simulink model "TCP40_ON_OFF"  (Simulink 8.1)
settings: Solver=ode45  StartTime=0.0  StopTime=150  RelTol=1e-3
settings Model: Creator=cslui  LastModifiedBy=tohoanglinh
settings OptimizationCC: BlockReduction=off  BooleanDataType=off  ExpressionDepthLimit=128
settings DebuggingCC: SaveWithParameterizedLinksMsg=none  SignalResolutionControl=TryResolveAllWithWarning  SolverPrmCheckMsg=none  MultiTaskDSMMsg=warning  MultiTaskCondExecSysMsg=none  FcnCallInpInsideContextMsg=EnableAllAsError  StrictBusMsg=None
settings HardwareCC: TargetUnknown=on
settings RTWCC: IncludeERTFirstTime=on

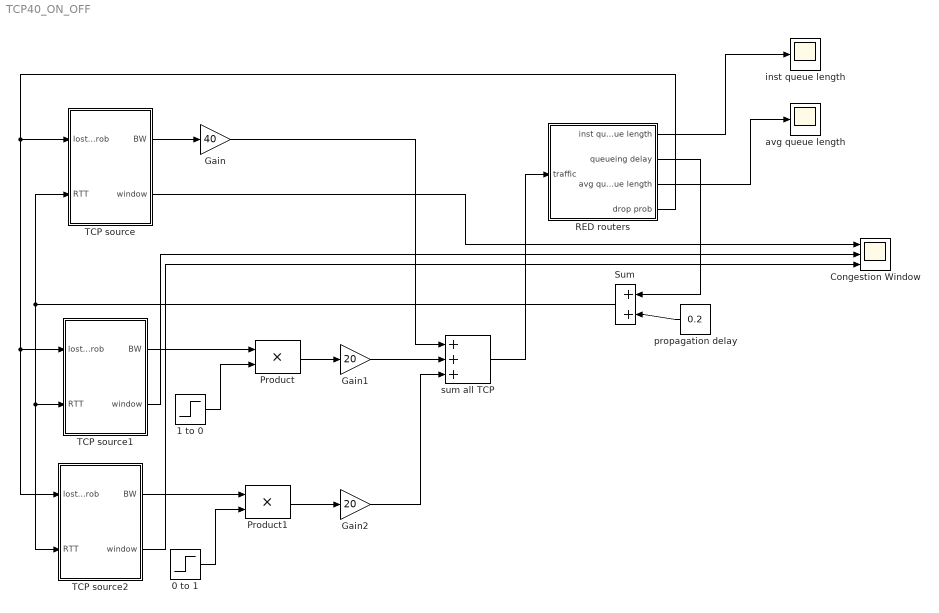
== system TCP40_ON_OFF ==
  0 to 1 : Step  Time=120  SampleTime=0
  1 to 0 : Step  Time=70  Before=1  After=0  SampleTime=0
  "Congestion Window " : Scope  NumInputPorts=3
      settings: YMin=0~-5~-5  YMax=30~5~5  SaveName=ScopeData2
  Gain : Gain  Gain=40  SaturateOnIntegerOverflow=on  OutDataTypeStr=Inherit: Same as input  ParamDataTypeStr=Inherit: Same as input
  Gain1 : Gain  Gain=20  SaturateOnIntegerOverflow=on  OutDataTypeStr=Inherit: Same as input  ParamDataTypeStr=Inherit: Same as input
  Gain2 : Gain  Gain=20  SaturateOnIntegerOverflow=on  OutDataTypeStr=Inherit: Same as input  ParamDataTypeStr=Inherit: Same as input
  Product : Product  SaturateOnIntegerOverflow=on  RndMeth=Zero  InputSameDT=on  OutDataTypeStr=Inherit: Same as first input
  Product1 : Product  SaturateOnIntegerOverflow=on  RndMeth=Zero  InputSameDT=on  OutDataTypeStr=Inherit: Same as first input
  RED routers : Subsystem  mask{C=1310}
      mask prompts: C "Router Capacity"
  Sum : Sum  Inputs=+|+  InputSameDT=on  OutDataTypeStr=Inherit: Same as first input
  TCP source : Subsystem
  TCP source1 : Subsystem
  TCP source2 : Subsystem
  avg queue length : Scope
      settings: YMin=0  YMax=800
  inst queue length : Scope
      settings: YMin=0  YMax=1000
  propagation delay : Constant  Value=0.2
  sum all TCP : Sum  Inputs=+|+|+  SaturateOnIntegerOverflow=on  InputSameDT=on  OutDataTypeStr=Inherit: Same as first input
  wires:
  TCP source/1(BW) -> Gain/1
  RED routers/2(queueing delay) -> Sum/1
  propagation delay/1 -> Sum/2
  Sum/1 -> TCP source/2(RTT), TCP source1/2(RTT), TCP source2/2(RTT)
  RED routers/4(drop prob) -> TCP source/1(lost prob), TCP source1/1(lost prob), TCP source2/1(lost prob)
  RED routers/1(inst queue length) -> inst queue length/1
  RED routers/3(avg queue length) -> avg queue length/1
  TCP source/2(window) -> "Congestion Window "/1
  TCP source1/1(BW) -> Product/1
  1 to 0/1 -> Product/2
  Product/1 -> Gain1/1
  TCP source2/1(BW) -> Product1/1
  0 to 1/1 -> Product1/2
  Product1/1 -> Gain2/1
  Gain/1 -> sum all TCP/1
  Gain2/1 -> sum all TCP/3
  sum all TCP/1 -> RED routers/1(traffic)
  Gain1/1 -> sum all TCP/2
  TCP source1/2(window) -> "Congestion Window "/2
  TCP source2/2(window) -> "Congestion Window "/3

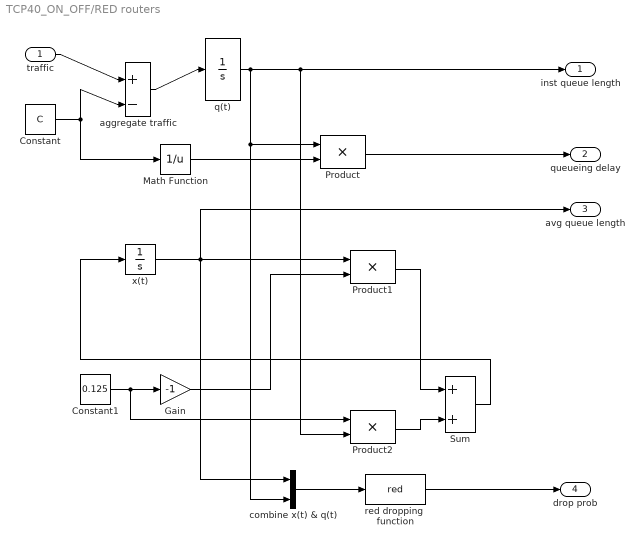
== system TCP40_ON_OFF/RED routers ==
  traffic : Inport
  Constant : Constant  Value=C
  Constant1 : Constant  Value=0.125
  Gain : Gain  Gain=-1  SaturateOnIntegerOverflow=on  OutDataTypeStr=Inherit: Same as input  ParamDataTypeStr=Inherit: Same as input
  Math Function : Math  Operator=reciprocal  SaturateOnIntegerOverflow=on
  Product : Product  SaturateOnIntegerOverflow=on  RndMeth=Zero  InputSameDT=on  OutDataTypeStr=Inherit: Same as first input
  Product1 : Product  SaturateOnIntegerOverflow=on  RndMeth=Zero  InputSameDT=on  OutDataTypeStr=Inherit: Same as first input
  Product2 : Product  SaturateOnIntegerOverflow=on  RndMeth=Zero  InputSameDT=on  OutDataTypeStr=Inherit: Same as first input
  Sum : Sum  SaturateOnIntegerOverflow=on  InputSameDT=on  OutDataTypeStr=Inherit: Same as first input
  "aggregate traffic " : Sum  Inputs=+|-  SaturateOnIntegerOverflow=on  InputSameDT=on  OutDataTypeStr=Inherit: Same as first input
  combine x(t) & q(t) : Mux  Inputs=2
  q(t) : Integrator  LimitOutput=on  UpperSaturationLimit=8000  LowerSaturationLimit=0
  red dropping  function : MATLABFcn  MATLABFcn=red  OutputSignalType=real
  x(t) : Integrator  LimitOutput=on  LowerSaturationLimit=0
  inst queue length : Outport
  queueing delay : Outport  Port=2
  avg queue length : Outport  Port=3
  drop prob : Outport  Port=4
  wires:
  traffic/1 -> "aggregate traffic "/1
  Constant/1 -> "aggregate traffic "/2, Math Function/1
  "aggregate traffic "/1 -> q(t)/1
  q(t)/1 -> inst queue length/1, Product2/2, Product/1, combine x(t) & q(t)/2
  Math Function/1 -> Product/2
  Product/1 -> queueing delay/1
  x(t)/1 -> Product1/1, avg queue length/1, combine x(t) & q(t)/1
  Constant1/1 -> Gain/1, Product2/1
  Gain/1 -> Product1/2
  Product1/1 -> Sum/1
  Product2/1 -> Sum/2
  Sum/1 -> x(t)/1
  combine x(t) & q(t)/1 -> red dropping  function/1
  red dropping  function/1 -> drop prob/1

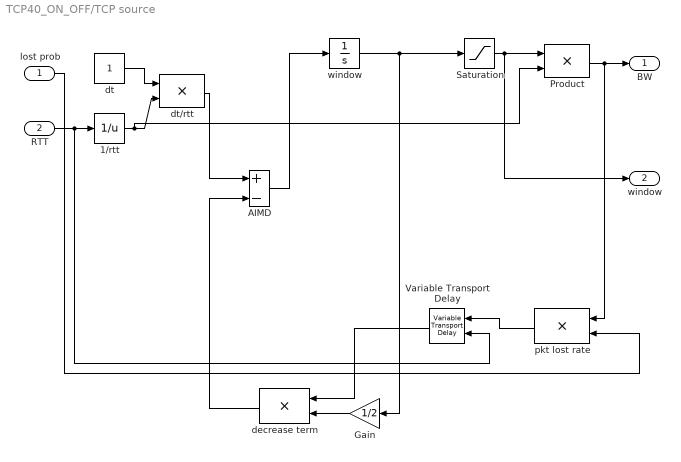
== system TCP40_ON_OFF/TCP source ==
  lost prob : Inport
  RTT : Inport  Port=2
  1/rtt : Math  Operator=reciprocal  SaturateOnIntegerOverflow=on
  AIMD : Sum  Inputs=+|-  SaturateOnIntegerOverflow=on  InputSameDT=on  OutDataTypeStr=Inherit: Same as first input
  Gain : Gain  Gain=1/2  SaturateOnIntegerOverflow=on  OutDataTypeStr=Inherit: Same as input  ParamDataTypeStr=Inherit: Same as input
  Product : Product  SaturateOnIntegerOverflow=on  RndMeth=Zero  InputSameDT=on  OutDataTypeStr=Inherit: Same as first input
  Saturation : Saturate  UpperLimit=500  LowerLimit=1
  Variable Transport Delay : VariableTransportDelay  MaximumDelay=10  MaximumPoints=20000  ZeroDelay=on
  decrease term : Product  SaturateOnIntegerOverflow=on  RndMeth=Zero  InputSameDT=on  OutDataTypeStr=Inherit: Same as first input
  dt : Constant
  dt/rtt : Product  SaturateOnIntegerOverflow=on  RndMeth=Zero  InputSameDT=on  OutDataTypeStr=Inherit: Same as first input
  pkt lost rate : Product  SaturateOnIntegerOverflow=on  RndMeth=Zero  InputSameDT=on  OutDataTypeStr=Inherit: Same as first input
  "window " : Integrator
  BW : Outport
  window : Outport  Port=2
  wires:
  "window "/1 -> Gain/1, Saturation/1
  Gain/1 -> decrease term/2
  decrease term/1 -> AIMD/2
  dt/1 -> dt/rtt/1
  1/rtt/1 -> dt/rtt/2, Product/2
  dt/rtt/1 -> AIMD/1
  AIMD/1 -> "window "/1
  RTT/1 -> 1/rtt/1, Variable Transport Delay/2
  Saturation/1 -> Product/1, window/1
  Product/1 -> BW/1, pkt lost rate/1
  lost prob/1 -> pkt lost rate/2
  pkt lost rate/1 -> Variable Transport Delay/1
  Variable Transport Delay/1 -> decrease term/1

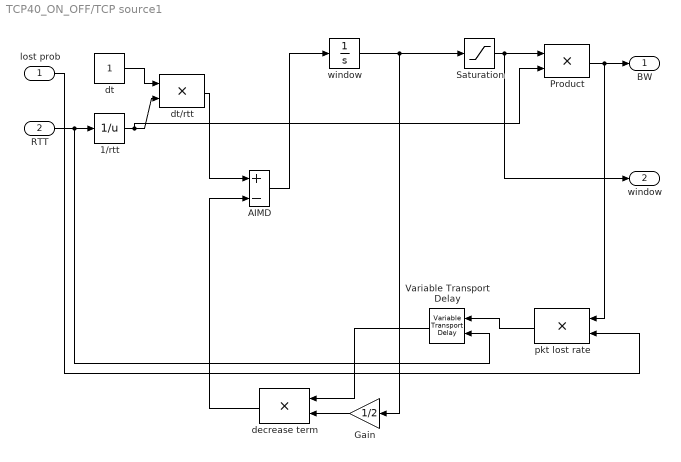
== system TCP40_ON_OFF/TCP source1 ==
  lost prob : Inport
  RTT : Inport  Port=2
  1/rtt : Math  Operator=reciprocal  SaturateOnIntegerOverflow=on
  AIMD : Sum  Inputs=+|-  SaturateOnIntegerOverflow=on  InputSameDT=on  OutDataTypeStr=Inherit: Same as first input
  Gain : Gain  Gain=1/2  SaturateOnIntegerOverflow=on  OutDataTypeStr=Inherit: Same as input  ParamDataTypeStr=Inherit: Same as input
  Product : Product  SaturateOnIntegerOverflow=on  RndMeth=Zero  InputSameDT=on  OutDataTypeStr=Inherit: Same as first input
  Saturation : Saturate  UpperLimit=500  LowerLimit=1
  Variable Transport Delay : VariableTransportDelay  MaximumDelay=10  MaximumPoints=20000  ZeroDelay=on
  decrease term : Product  SaturateOnIntegerOverflow=on  RndMeth=Zero  InputSameDT=on  OutDataTypeStr=Inherit: Same as first input
  dt : Constant
  dt/rtt : Product  SaturateOnIntegerOverflow=on  RndMeth=Zero  InputSameDT=on  OutDataTypeStr=Inherit: Same as first input
  pkt lost rate : Product  SaturateOnIntegerOverflow=on  RndMeth=Zero  InputSameDT=on  OutDataTypeStr=Inherit: Same as first input
  "window " : Integrator
  BW : Outport
  window : Outport  Port=2
  wires:
  "window "/1 -> Gain/1, Saturation/1
  Gain/1 -> decrease term/2
  decrease term/1 -> AIMD/2
  dt/1 -> dt/rtt/1
  1/rtt/1 -> dt/rtt/2, Product/2
  dt/rtt/1 -> AIMD/1
  AIMD/1 -> "window "/1
  RTT/1 -> 1/rtt/1, Variable Transport Delay/2
  Saturation/1 -> Product/1, window/1
  Product/1 -> BW/1, pkt lost rate/1
  lost prob/1 -> pkt lost rate/2
  pkt lost rate/1 -> Variable Transport Delay/1
  Variable Transport Delay/1 -> decrease term/1

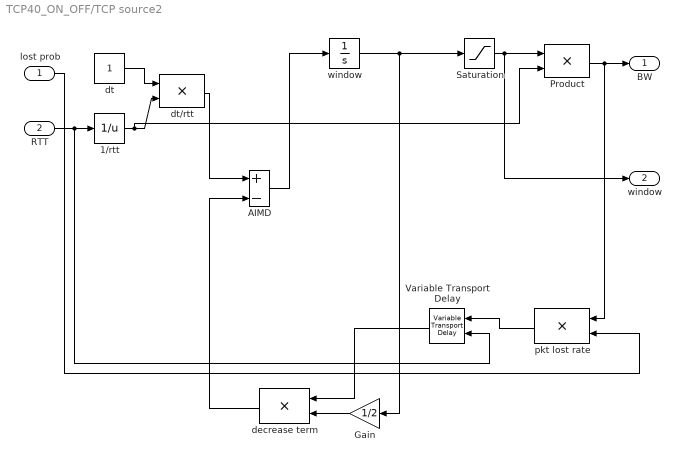
== system TCP40_ON_OFF/TCP source2 ==
  lost prob : Inport
  RTT : Inport  Port=2
  1/rtt : Math  Operator=reciprocal  SaturateOnIntegerOverflow=on
  AIMD : Sum  Inputs=+|-  SaturateOnIntegerOverflow=on  InputSameDT=on  OutDataTypeStr=Inherit: Same as first input
  Gain : Gain  Gain=1/2  SaturateOnIntegerOverflow=on  OutDataTypeStr=Inherit: Same as input  ParamDataTypeStr=Inherit: Same as input
  Product : Product  SaturateOnIntegerOverflow=on  RndMeth=Zero  InputSameDT=on  OutDataTypeStr=Inherit: Same as first input
  Saturation : Saturate  UpperLimit=500  LowerLimit=1
  Variable Transport Delay : VariableTransportDelay  MaximumDelay=10  MaximumPoints=20000  ZeroDelay=on
  decrease term : Product  SaturateOnIntegerOverflow=on  RndMeth=Zero  InputSameDT=on  OutDataTypeStr=Inherit: Same as first input
  dt : Constant
  dt/rtt : Product  SaturateOnIntegerOverflow=on  RndMeth=Zero  InputSameDT=on  OutDataTypeStr=Inherit: Same as first input
  pkt lost rate : Product  SaturateOnIntegerOverflow=on  RndMeth=Zero  InputSameDT=on  OutDataTypeStr=Inherit: Same as first input
  "window " : Integrator
  BW : Outport
  window : Outport  Port=2
  wires:
  "window "/1 -> Gain/1, Saturation/1
  Gain/1 -> decrease term/2
  decrease term/1 -> AIMD/2
  dt/1 -> dt/rtt/1
  1/rtt/1 -> dt/rtt/2, Product/2
  dt/rtt/1 -> AIMD/1
  AIMD/1 -> "window "/1
  RTT/1 -> 1/rtt/1, Variable Transport Delay/2
  Saturation/1 -> Product/1, window/1
  Product/1 -> BW/1, pkt lost rate/1
  lost prob/1 -> pkt lost rate/2
  pkt lost rate/1 -> Variable Transport Delay/1
  Variable Transport Delay/1 -> decrease term/1
